simulink model "wheeled_balancer_model_simscape"  (R2024b)
settings: Solver=VariableStepAuto  StartTime=0.0  StopTime=3  FixedStep=0.001  MaxStep=0.0001  RelTol=1e-3  AbsTol=1e-3  EnableMultiTasking=on
StartFcn:
  | wheeled_balancer_model_simscape
values from neighbouring files (symbols this model uses):
  A = double(subs(Api,[g,M,m,b,l,I],[g_real,M_real,m_real,b_real,     l_real,I_real]))    [Scratchwork_cart.m]    (also in Scratchwork_pendulums.m = [0 1; a/l 0]; wheeled_balancer_model_simscape_script.m = double(subs(Asym,[g_sym,m_c_sym,m_sym,mu_c_sym,l_sym,J_sym,r)
  B = double(subs(Bpi,[g,M,m,b,l,I],[g_real,M_real,m_real,b_real,     l_real,I_real]))    [Scratchwork_cart.m]    (also in Scratchwork_pendulums.m = [0; 1/(m*l^2)]; wheeled_balancer_model_simscape_script.m = double(subs(Bsym,[g_sym,m_c_sym,m_sym,mu_c_sym,l_sym,J_sym,r)
  C = [1 0 0 0; 0 0 1 0]    [Scratchwork_cart.m]    (also in Scratchwork_pendulums.m = [1 0]; wheeled_balancer_model_simscape_script.m = [1 0 0 0; 0 0 0 1])
  C2 = [1 0]    [wheeled_balancer_model_simscape_script.m]
  g = 9.81    [wheeled_balancer_model_simscape_script.m]
  J = (I_motor + I_bump + I_batt + I_cb)    (= 0.000441007536814)    [wheeled_balancer_model_simscape_script.m]
  K = acker(A,B,p)    [Scratchwork_cart.m]    (also in Scratchwork_pendulums.m = acker(A,B,poles); wheeled_balancer_model_simscape_script.m = acker(Abar, Bbar, pc_control), Ks = K(1:end-1))
  Ki = K(end)    [wheeled_balancer_model_simscape_script.m]
  Ks = K(1:end-1), Ki = K(end),    [wheeled_balancer_model_simscape_script.m]
  L = place(A',C',pc_observer)'    [wheeled_balancer_model_simscape_script.m]
  l = .1    (= 0.1)    [Scratchwork_pendulums.m]    (also in wheeled_balancer_model_simscape_script.m = CM_rot)
  m = 1    [Scratchwork_pendulums.m]    (also in wheeled_balancer_model_simscape_script.m = 0.2983)
  m_c = (m_wheels)    (= 0.0397)    [wheeled_balancer_model_simscape_script.m]
  mu_c = 0.02    [wheeled_balancer_model_simscape_script.m]
  r = 0.01    [Scratchwork_pendulums.m]    (also in wheeled_balancer_model_simscape_script.m = 0.04)
  T = 1/100    (= 0.01)    [wheeled_balancer_model_simscape_script.m]
  theta_init = 0    [wheeled_balancer_model_simscape_script.m]
undefined symbols (not defined in the file or in its folder): Cd, G, H, X, Y, Z
libraries: sm_lib x8, nesl_utility x6
settings Model: Creator=teowi  LastModifiedBy=teowi
settings SolverCC: AutoScaleAbsTol=off  AlgebraicLoopSolver=TrustRegion  MaxZcPerStep=1
settings DataIOCC: LimitDataPoints=on  MaxDataPoints=10000
settings OptimizationCC: ReuseModelBlockBuffer=off  LifeSpan=inf
settings DebuggingCC: UnconnectedInputMsg=warning  UnconnectedOutputMsg=warning  UnconnectedLineMsg=warning  AllowSymbolicDim=off  SubsystemReferenceDiagnosticForUnitTest=warning  SFUnexpectedBacktrackingDiag=warning  SFNoUnconditionalDefaultTransitionDiag=warning  SFExecutionAtInitializationDiag=none  ArithmeticOperatorsInVariantConditions=warning
settings ModelReferenceCC: EnableRefExpFcnMdlSchedulingChecks=on
settings SFSimCC: SimUseLocalCustomCode=off  CustomCodeUndefinedFunction=UseInterfaceOnly
settings RTWCC: RTWUseLocalCustomCode=off  GPUComputeCapability=3.5  DLArmComputeVersion=19.05
settings CodeAppCC: StateflowObjectComments=on
settings GRTTargetCC: TargetLangStandard=C89/C90 (ANSI)
settings ConfigComp: CovMetricSettings=dw  CovSaveCumulativeToWorkspaceVar=on  CovSaveSingleToWorkspaceVar=on  CovExternalEMLEnable=off  CovSFcnEnable=off
settings SimscapeCC: SimscapeLogType=all  SimscapeLogSimulationStatistics=on  SimscapeLogDataHistory=10000

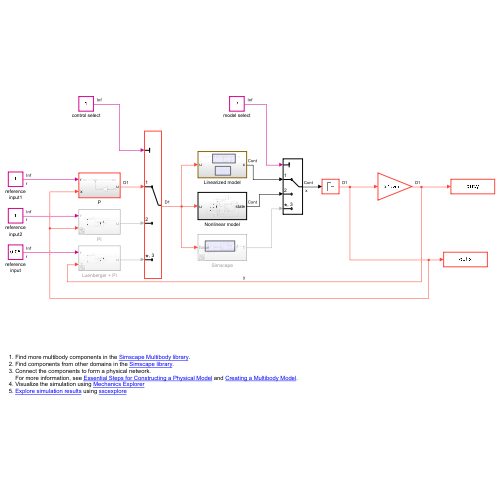
[thumbnail: Simulink's stored preview of the top-level diagram]
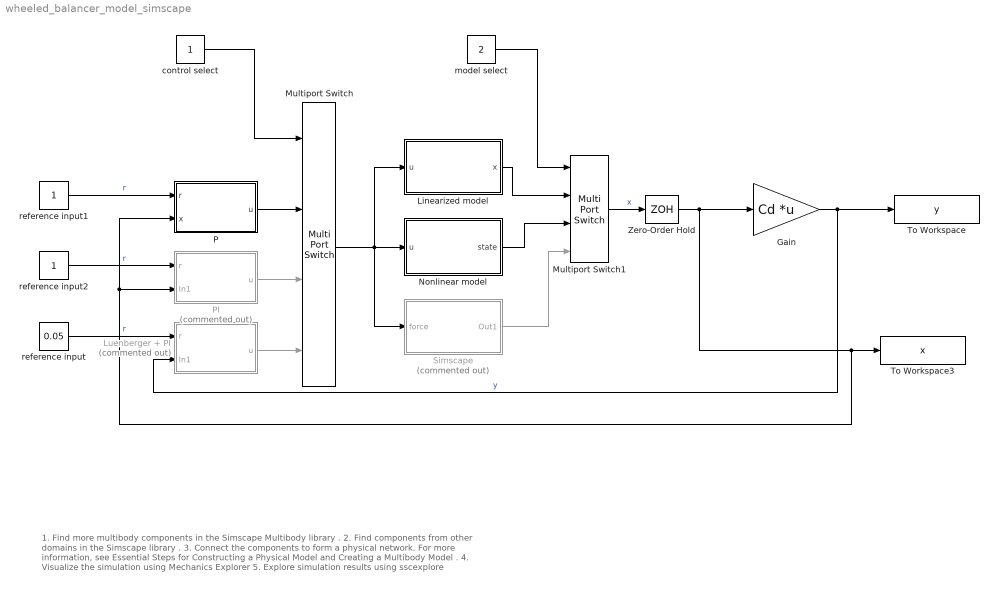
== system wheeled_balancer_model_simscape ==
  note: 1. Find more multibody components in the Simscape Multibody library .
      | 2. Find components from other domains in the Simscape library .
      | 3. Connect the components to form a physical network.
      | For more information, see Essential Steps for Constructing a Physical Model and Creating a Multibody Model .
      | 4. Visualize the simulation using Mechanics Explorer
      | 5. Explore simulation results using sscexplore
  Gain : Gain  Gain=Cd  Multiplication=Matrix(K*u) (u vector)
  Linearized model : Subsystem
  Luenberger + PI : Subsystem  Commented=on
  Multiport Switch : MultiPortSwitch  SaturateOnIntegerOverflow=off  InputSameDT=off
  Multiport Switch1 : MultiPortSwitch  SaturateOnIntegerOverflow=off  InputSameDT=off
  Nonlinear model : Subsystem
  P : Subsystem
  PI : Subsystem  Commented=on
  Simscape : Subsystem  Commented=on
  To Workspace : ToWorkspace  VariableName=y  SaveFormat=Timeseries  SampleTime=-1
  To Workspace3 : ToWorkspace  VariableName=x  SaveFormat=Timeseries  SampleTime=-1
  Zero-Order Hold : ZeroOrderHold  SampleTime=T
  control select : Constant
  model select : Constant  Value=2
  reference input : Constant  Value=0.05
  reference input1 : Constant
  reference input2 : Constant
  wires:
  Gain/1 -> To Workspace/1, Luenberger + PI/2(In1)  "y"
  Multiport Switch1/1 -> Zero-Order Hold/1  "x"
  control select/1 -> Multiport Switch/1
  Luenberger + PI/1(u) -> Multiport Switch/4
  reference input/1 -> Luenberger + PI/1(r)  "r"
  PI/1(u) -> Multiport Switch/3
  P/1(u) -> Multiport Switch/2
  reference input1/1 -> P/1(r)  "r"
  reference input2/1 -> PI/1(r)  "r"
  Multiport Switch/1 -> Simscape/1(force), Nonlinear model/1(u), Linearized model/1(u)
  Simscape/1(Out1) -> Multiport Switch1/4
  Linearized model/1(x) -> Multiport Switch1/2
  model select/1 -> Multiport Switch1/1
  Nonlinear model/1(state) -> Multiport Switch1/3
  Zero-Order Hold/1 -> To Workspace3/1, PI/2(In1), P/2(x), Gain/1

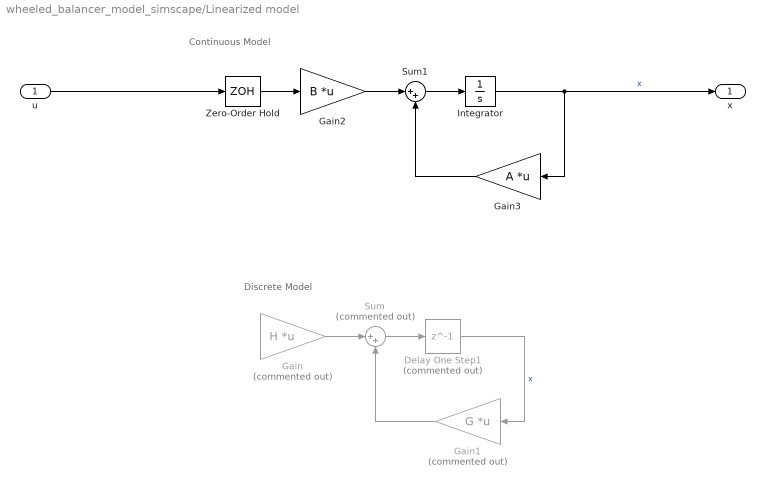
== system wheeled_balancer_model_simscape/Linearized model ==
  note: Discrete Model
  note: Continuous Model
  u : Inport
  Delay One Step1 : Delay  Commented=on  DelayLength=1  SampleTime=T
  Gain : Gain  Commented=on  Gain=H  Multiplication=Matrix(K*u) (u vector)
  Gain1 : Gain  Commented=on  Gain=G  Multiplication=Matrix(K*u) (u vector)
  Gain2 : Gain  Gain=B  Multiplication=Matrix(K*u) (u vector)
  Gain3 : Gain  Gain=A  Multiplication=Matrix(K*u) (u vector)
  Integrator : Integrator
  Sum : Sum  Commented=on  Inputs=|++
  Sum1 : Sum  Inputs=|++
  Zero-Order Hold : ZeroOrderHold  SampleTime=-1
  x : Outport
  wires:
  Sum/1 -> Delay One Step1/1
  Delay One Step1/1 -> Gain1/1  "x"
  Gain/1 -> Sum/1
  Gain1/1 -> Sum/2
  Integrator/1 -> Gain3/1, x/1  "x"
  Gain2/1 -> Sum1/1
  Sum1/1 -> Integrator/1
  Gain3/1 -> Sum1/2
  Zero-Order Hold/1 -> Gain2/1
  u/1 -> Zero-Order Hold/1

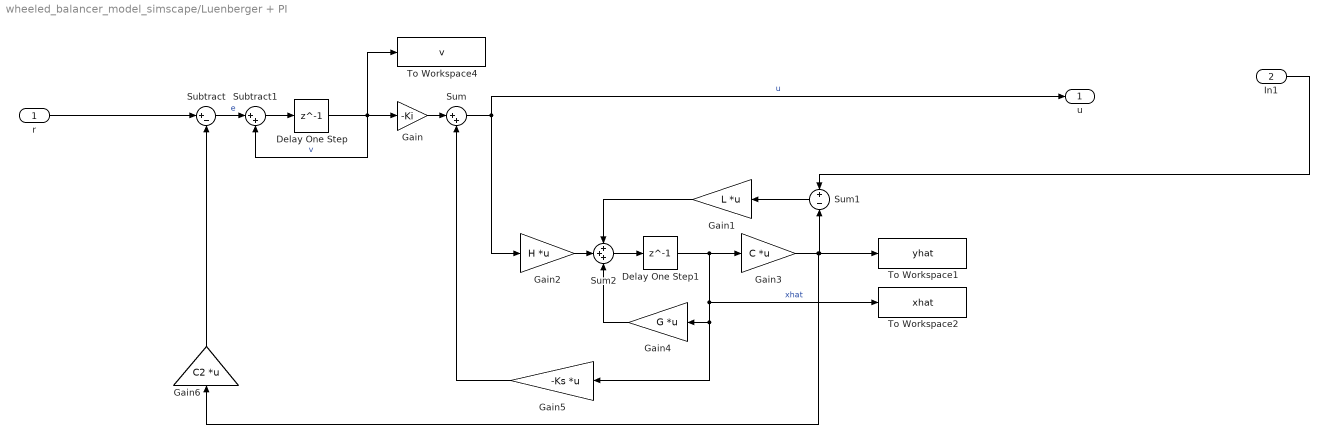
== system wheeled_balancer_model_simscape/Luenberger + PI ==
  r : Inport
  In1 : Inport  Port=2
  Delay One Step : Delay  DelayLength=1  SampleTime=T
  Delay One Step1 : Delay  DelayLength=1  SampleTime=T
  Gain : Gain  Gain=-Ki
  Gain1 : Gain  Gain=L  Multiplication=Matrix(K*u) (u vector)
  Gain2 : Gain  Gain=H  Multiplication=Matrix(K*u) (u vector)
  Gain3 : Gain  Gain=C  Multiplication=Matrix(K*u) (u vector)
  Gain4 : Gain  Gain=G  Multiplication=Matrix(K*u) (u vector)
  Gain5 : Gain  Gain=-Ks  Multiplication=Matrix(K*u) (u vector)
  Gain6 : Gain  Gain=C2  Multiplication=Matrix(K*u) (u vector)
  Subtract : Sum  Inputs=|+-
  Subtract1 : Sum  Inputs=|++
  Sum : Sum  Inputs=|++
  Sum1 : Sum  Inputs=+|-
  Sum2 : Sum  Inputs=+++
  To Workspace1 : ToWorkspace  VariableName=yhat  SaveFormat=Timeseries  SampleTime=-1
  To Workspace2 : ToWorkspace  VariableName=xhat  SaveFormat=Timeseries  SampleTime=-1
  To Workspace4 : ToWorkspace  VariableName=v  SaveFormat=Timeseries  SampleTime=-1
  u : Outport
  wires:
  Delay One Step1/1 -> Gain4/1, Gain5/1, To Workspace2/1, Gain3/1  "xhat"
  Sum/1 -> u/1, Gain2/1  "u"
  r/1 -> Subtract/1
  Delay One Step/1 -> To Workspace4/1, Gain/1, Subtract1/2  "v"
  Gain5/1 -> Sum/2
  Subtract/1 -> Subtract1/1  "e"
  Gain/1 -> Sum/1
  Gain1/1 -> Sum2/1
  Gain3/1 -> To Workspace1/1, Sum1/2, Gain6/1
  Gain2/1 -> Sum2/2
  Sum1/1 -> Gain1/1
  Gain6/1 -> Subtract/2
  Subtract1/1 -> Delay One Step/1
  Gain4/1 -> Sum2/3
  Sum2/1 -> Delay One Step1/1
  In1/1 -> Sum1/1

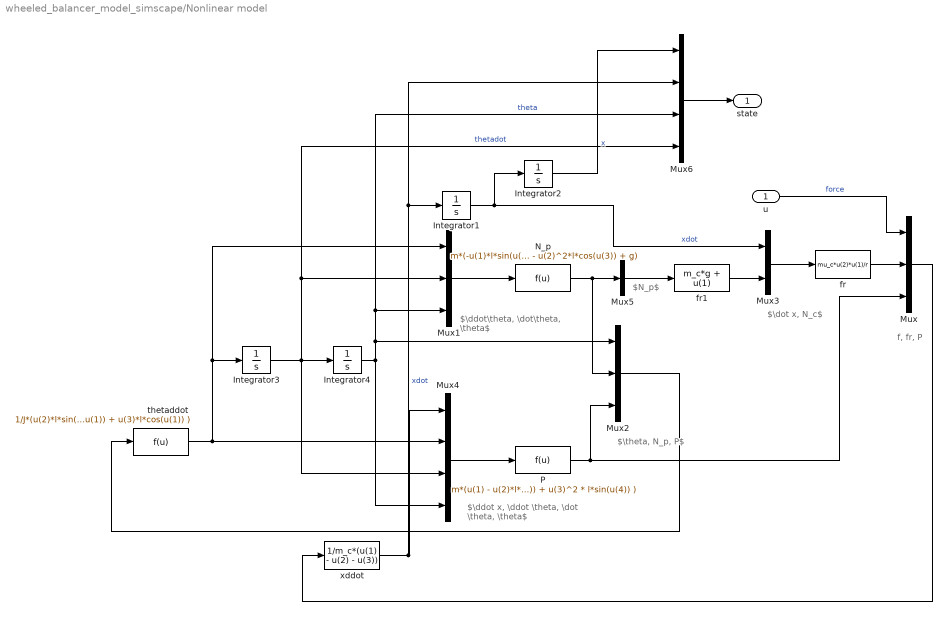
== system wheeled_balancer_model_simscape/Nonlinear model ==
  note: f, fr, P
  note: $\theta, N_p, P$
  note: $\dot x, N_c$
  note: $N_p$
  note: $\ddot\theta, \dot\theta, \theta$
  note: $\ddot x, \ddot \theta, \dot \theta, \theta$
  u : Inport
  Integrator1 : Integrator
  Integrator2 : Integrator
  Integrator3 : Integrator
  Integrator4 : Integrator  InitialCondition=theta_init
  Mux : Mux  Inputs=3
  Mux1 : Mux  Inputs=3
  Mux2 : Mux  Inputs=3
  Mux3 : Mux  Inputs=2
  Mux4 : Mux
  Mux5 : Mux  Inputs=1
  Mux6 : Mux
  N_p : Fcn  Expr=m*(-u(1)*l*sin(u(3)) - u(2)^2*l*cos(u(3)) + g)
  P : Fcn  Expr=m*(u(1) - u(2)*l*cos(u(4)) + u(3)^2 * l*sin(u(4)) )
  fr : Fcn  Expr=mu_c*u(2)*u(1)/r
  fr1 : Fcn  Expr=m_c*g + u(1)
  thetaddot : Fcn  Expr=1/J*(u(2)*l*sin(u(1)) + u(3)*l*cos(u(1)) )
  xddot : Fcn  Expr=1/m_c*(u(1) - u(2) - u(3))
  state : Outport
  wires:
  Mux2/1 -> thetaddot/1
  Integrator1/1 -> Integrator2/1, Mux3/1  "xdot"
  xddot/1 -> Mux6/2, Integrator1/1, Mux4/1  "xdot"
  thetaddot/1 -> Mux1/1, Integrator3/1, Mux4/2
  Integrator4/1 -> Mux2/1, Mux6/3, Mux1/3, Mux4/4  "theta"
  Integrator3/1 -> Mux4/3, Integrator4/1, Mux6/4, Mux1/2  "thetadot"
  Mux4/1 -> P/1
  Mux1/1 -> N_p/1
  N_p/1 -> Mux5/1, Mux2/2
  fr1/1 -> Mux3/2
  P/1 -> Mux/3, Mux2/3
  Mux5/1 -> fr1/1
  Mux/1 -> xddot/1
  Mux3/1 -> fr/1
  u/1 -> Mux/1  "force"
  fr/1 -> Mux/2
  Integrator2/1 -> Mux6/1  "x"
  Mux6/1 -> state/1

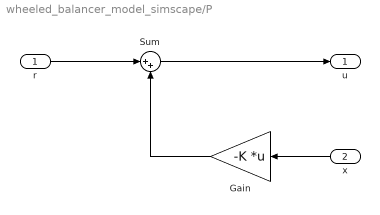
== system wheeled_balancer_model_simscape/P ==
  r : Inport
  x : Inport  Port=2
  Gain : Gain  Gain=-K  Multiplication=Matrix(K*u) (u vector)
  Sum : Sum  Inputs=|++
  u : Outport
  wires:
  r/1 -> Sum/1
  x/1 -> Gain/1
  Gain/1 -> Sum/2
  Sum/1 -> u/1

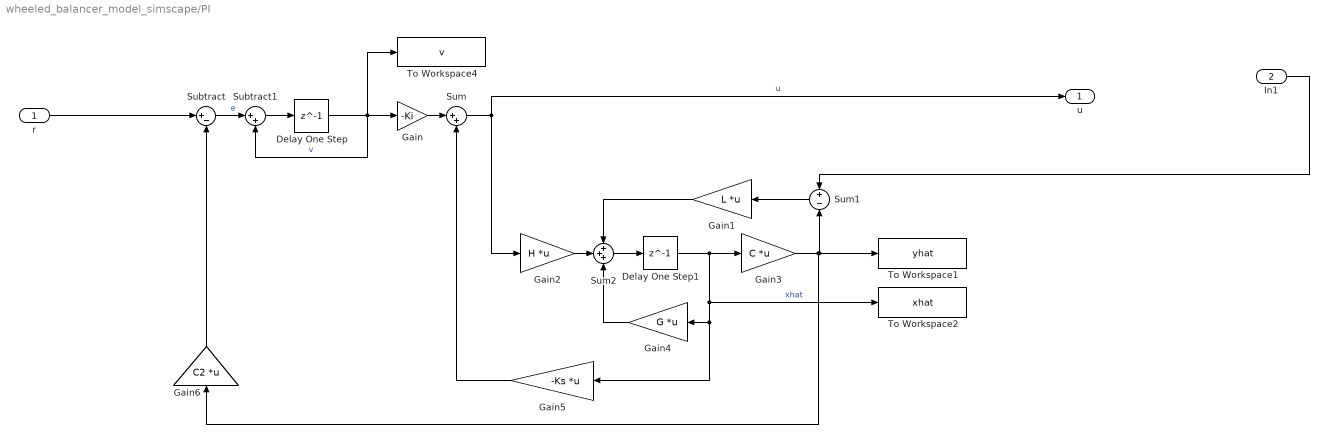
== system wheeled_balancer_model_simscape/PI ==
  r : Inport
  In1 : Inport  Port=2
  Delay One Step : Delay  DelayLength=1  SampleTime=T
  Delay One Step1 : Delay  DelayLength=1  SampleTime=T
  Gain : Gain  Gain=-Ki
  Gain1 : Gain  Gain=L  Multiplication=Matrix(K*u) (u vector)
  Gain2 : Gain  Gain=H  Multiplication=Matrix(K*u) (u vector)
  Gain3 : Gain  Gain=C  Multiplication=Matrix(K*u) (u vector)
  Gain4 : Gain  Gain=G  Multiplication=Matrix(K*u) (u vector)
  Gain5 : Gain  Gain=-Ks  Multiplication=Matrix(K*u) (u vector)
  Gain6 : Gain  Gain=C2  Multiplication=Matrix(K*u) (u vector)
  Subtract : Sum  Inputs=|+-
  Subtract1 : Sum  Inputs=|++
  Sum : Sum  Inputs=|++
  Sum1 : Sum  Inputs=+|-
  Sum2 : Sum  Inputs=+++
  To Workspace1 : ToWorkspace  VariableName=yhat  SaveFormat=Timeseries  SampleTime=-1
  To Workspace2 : ToWorkspace  VariableName=xhat  SaveFormat=Timeseries  SampleTime=-1
  To Workspace4 : ToWorkspace  VariableName=v  SaveFormat=Timeseries  SampleTime=-1
  u : Outport
  wires:
  Delay One Step1/1 -> Gain4/1, Gain5/1, To Workspace2/1, Gain3/1  "xhat"
  Sum/1 -> u/1, Gain2/1  "u"
  r/1 -> Subtract/1
  Delay One Step/1 -> To Workspace4/1, Gain/1, Subtract1/2  "v"
  Gain5/1 -> Sum/2
  Subtract/1 -> Subtract1/1  "e"
  Gain/1 -> Sum/1
  Gain1/1 -> Sum2/1
  Gain3/1 -> To Workspace1/1, Sum1/2, Gain6/1
  Gain2/1 -> Sum2/2
  Sum1/1 -> Gain1/1
  Gain6/1 -> Subtract/2
  Subtract1/1 -> Delay One Step/1
  Gain4/1 -> Sum2/3
  Sum2/1 -> Delay One Step1/1
  In1/1 -> Sum1/1

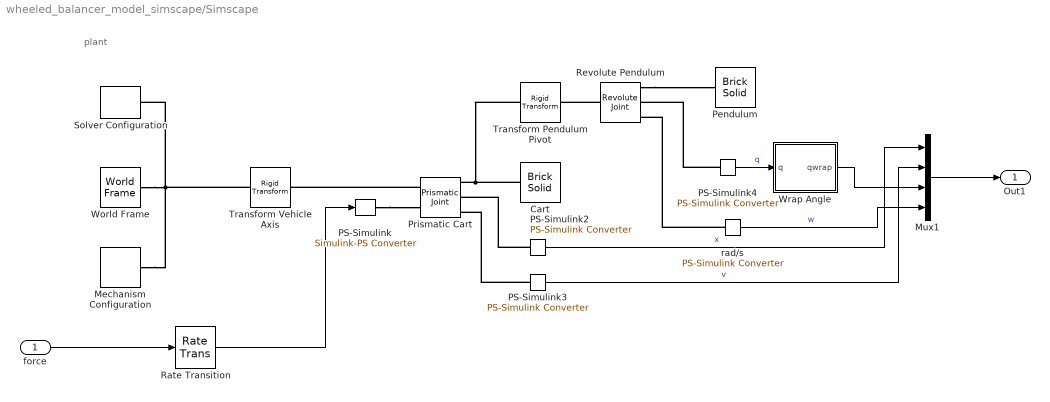
== system wheeled_balancer_model_simscape/Simscape ==
  note: plant
  force : Inport
  Cart : sm_lib/Body Elements/Brick Solid  BrickDimensions=[0.02 0.04 0.06]  BrickDimensionsUnits=m  ExportEntireGeometry=off  InertiaType=PointMass  BasedOnType=Density  Density=1000  DensityUnits=kg/m^3  Mass=m_c  MassUnits=kg  CenterOfMass=[0 0 0]  CenterOfMassUnits=m  MomentsOfInertia=[1 1 1]  MomentsOfInertiaUnits=kg*m^2  ProductsOfInertia=[0 0 0]  ProductsOfInertiaUnits=kg*m^2  GraphicType=FromGeometry  MarkerShape=Sphere  MarkerSize=10  GraphicVisPropType=SimpleVisualProperties  GraphicDiffuseColor=[0.8 0.45 0]  GraphicOpacity=1.0  GraphicSpecularColor=[0.5 0.5 0.5 1.0]  GraphicAmbientColor=[0.15 0.15 0.15 1.0]  GraphicEmissiveColor=[0.0 0.0 0.0 1.0]  GraphicShininess=75  DoExposeReferenceFrame=on  SerializedFrames=<Frames/>
  Mechanism Configuration : sm_lib/Utilities/Mechanism Configuration  UniformGravity=Constant  GravityVector=[0 0 -g]  GravityVectorUnits=m/s^2  LinearizationDelta=0.001  JointModeTransitionNonlinearIterations=2
  Mux1 : Mux
  PS-Simulink : nesl_utility/Simulink-PS Converter  PhysicalDomain=network_engine_domain  SubClassName=ps_input  LeftPortType=input  RightPortType=output  PseudoPeriodic=off  Frequencies=[]  NoiseDistribution=none  NoiseParameters=[]  Unit=N  AffineConversion=off  FilteringAndDerivatives=provide  SimscapeFilterOrder=1  InputFilterTimeConstant=0.001  UdotUserProvided=0
  PS-Simulink2 : nesl_utility/PS-Simulink Converter  PhysicalDomain=network_engine_domain  SubClassName=ps_output  LeftPortType=input  RightPortType=output  PseudoPeriodic=off  Frequencies=[]  VectorFormat=inherit  Unit=m  AffineConversion=off
  PS-Simulink3 : nesl_utility/PS-Simulink Converter  PhysicalDomain=network_engine_domain  SubClassName=ps_output  LeftPortType=input  RightPortType=output  PseudoPeriodic=off  Frequencies=[]  VectorFormat=inherit  Unit=m/s  AffineConversion=off
  PS-Simulink4 : nesl_utility/PS-Simulink Converter  PhysicalDomain=network_engine_domain  SubClassName=ps_output  LeftPortType=input  RightPortType=output  PseudoPeriodic=off  Frequencies=[]  VectorFormat=inherit  Unit=rad  AffineConversion=off
  Pendulum : sm_lib/Body Elements/Brick Solid  BrickDimensions=[l*2 0.04 0.02]  BrickDimensionsUnits=m  ExportEntireGeometry=off  InertiaType=PointMass  BasedOnType=Density  Density=1000  DensityUnits=kg/m^3  Mass=m  MassUnits=kg  CenterOfMass=[0 0 0]  CenterOfMassUnits=m  MomentsOfInertia=[1 1 1]  MomentsOfInertiaUnits=kg*m^2  ProductsOfInertia=[0 0 0]  ProductsOfInertiaUnits=kg*m^2  GraphicType=FromGeometry  MarkerShape=Sphere  MarkerSize=10  GraphicVisPropType=SimpleVisualProperties  GraphicDiffuseColor=[0.25 0.4 0.7]  GraphicOpacity=1  GraphicSpecularColor=[0.5 0.5 0.5 1.0]  GraphicAmbientColor=[0.15 0.15 0.15 1.0]  GraphicEmissiveColor=[0.0 0.0 0.0 1.0]  GraphicShininess=75  DoExposeReferenceFrame=off  SerializedFrames=<Frames><Frame><Id>Frame1</Id><Value><Name>B</Name><Origin><Source>GeometricFeature</Source><FeatureName>+x surface</FeatureName></Origin><PrimaryAxis><DefinedDirection>+Z</DefinedDirection><Source>ReferenceFrame</Source><SourceDirection>+Z</SourceDirection><FeatureName></FeatureName></PrimaryAxis><SecondaryAxis><DefinedDirection>+X</DefinedDirection><Source>ReferenceFrame</Source><SourceDirection>+X</SourceDirection><FeatureName></FeatureName></SecondaryAxis></Value></Frame></Frames>
  Prismatic Cart : sm_lib/Joints/Prismatic Joint  JointMode=Normal  CompositeWrenchDir=FollowerOnBase  CompositeWrenchFrame=BaseFrame  SenseConstraintForce=off  SenseConstraintTorque=off  SenseTotalForce=off  SenseTotalTorque=off  PositionTargetSpecify=off  PositionTargetPriority=High  PositionTargetValue=0  PositionTargetValueUnits=m  VelocityTargetSpecify=off  VelocityTargetPriority=High  VelocityTargetValue=0  VelocityTargetValueUnits=m/s  EquilibriumPosition=0  EquilibriumPositionUnits=m  SpringStiffness=0  SpringStiffnessUnits=N/m  DampingCoefficient=mu_c*(m+m_c)*g/r  DampingCoefficientUnits=N/(m/s)  LowerLimitSpecify=off  LowerLimitBound=-1  LowerLimitBoundUnits=m  LowerLimitStiffness=1e6  LowerLimitStiffnessUnits=N/m  LowerLimitDamping=1e3  LowerLimitDampingUnits=N/(m/s)  LowerLimitTransitionRegionWidth=1e-4  LowerLimitTransitionRegionWidthUnits=m  UpperLimitSpecify=off  UpperLimitBound=1  UpperLimitBoundUnits=m  UpperLimitStiffness=1e6  UpperLimitStiffnessUnits=N/m  UpperLimitDamping=1e3  UpperLimitDampingUnits=N/(m/s)  UpperLimitTransitionRegionWidth=1e-4  UpperLimitTransitionRegionWidthUnits=m  TorqueActuationMode=InputTorque  MotionActuationMode=ComputedMotion  SensePosition=on  SenseVelocity=on  SenseAcceleration=off  SenseTorqueForce=off  SenseLowerLimitTorqueForce=off  SenseUpperLimitTorqueForce=off
  Rate Transition : RateTransition
  Revolute Pendulum : sm_lib/Joints/Revolute Joint  JointMode=Normal  CompositeWrenchDir=FollowerOnBase  CompositeWrenchFrame=BaseFrame  SenseConstraintForce=off  SenseConstraintTorque=off  SenseTotalForce=off  SenseTotalTorque=off  PositionTargetSpecify=off  PositionTargetPriority=High  PositionTargetValue=0  PositionTargetValueUnits=deg  VelocityTargetSpecify=off  VelocityTargetPriority=High  VelocityTargetValue=0  VelocityTargetValueUnits=deg/s  EquilibriumPosition=0  EquilibriumPositionUnits=deg  SpringStiffness=0  SpringStiffnessUnits=N*m/deg  DampingCoefficient=0  DampingCoefficientUnits=N*m/(deg/s)  LowerLimitSpecify=off  LowerLimitBound=-90  LowerLimitBoundUnits=deg  LowerLimitStiffness=1e4  LowerLimitStiffnessUnits=N*m/deg  LowerLimitDamping=10  LowerLimitDampingUnits=N*m/(deg/s)  LowerLimitTransitionRegionWidth=0.1  LowerLimitTransitionRegionWidthUnits=deg  UpperLimitSpecify=off  UpperLimitBound=90  UpperLimitBoundUnits=deg  UpperLimitStiffness=1e4  UpperLimitStiffnessUnits=N*m/deg  UpperLimitDamping=10  UpperLimitDampingUnits=N*m/(deg/s)  UpperLimitTransitionRegionWidth=0.1  UpperLimitTransitionRegionWidthUnits=deg  TorqueActuationMode=NoTorque  MotionActuationMode=ComputedMotion  SensePosition=on  SenseVelocity=on  SenseAcceleration=off  SenseTorqueForce=off  SenseLowerLimitTorqueForce=off  SenseUpperLimitTorqueForce=off
  Solver Configuration : nesl_utility/Solver Configuration  PhysicalDomain=network_engine_domain  SubClassName=solver  LeftPortType=input  RightPortType=generic  Tones=[]  Harmonics=[]  SimulateNoise=off  Profile=off  UseLocalSampling=off  EnableSwitchedLinearOptims=on  FrequencyDomain=off  UseCCode=off  RelTol=0.001  AbsTol=1e-06  MinStep=1e-09  ToWorkspace=off  RevertToSquareIcSolve=off  NumHomotopyIterations=100  PhasorMode=off  PhasorModeNumHarmonics=1  ConsistencySolver=NEWTON_XTOL_AFTER_FTOL  IndexReductionMethod=DerivativeReplacement  DoDC=off  ResidualTolerance=1e-09  ConsistencyTolSource=GLOBAL  ConsistencyAbsTol=0.001  ConsistencyRelTol=0.001  ConsistencyTolFactor=0.001  UseLocalSolver=off  LocalSolverChoice=NE_BACKWARD_EULER_ADVANCER  ResolveIndetEquations=on  FunctionEvalNumThread=1  LocalSolverSampleTime=0.0001  DoFixedCost=off  MaxNonlinIter=3  MaxModeIter=2  ComputeImpulses=off  ImpulseIterations=2  LinearAlgebra=Sparse  LinearAlgebraNumThread=0  EquationFormulation=NE_TIME_EF  DelaysMemoryBudget=1024  AutomaticFiltering=on  FilteringTimeConstant=0.001  PartitionStorageMethod=AS_NEEDED  PartitionMemoryBudget=1024  PartitionMethod=FAST  MultibodyUseLocalSolver=off  MultibodyLocalSolverChoice=ODE1  MultibodyLocalSolverSampleTime=0.001
  Transform Pendulum Pivot : sm_lib/Frames and Transforms/Rigid Transform  RotationMethod=StandardAxis  FollAlignAxisA=+X  BaseAlignAxisA=+Y  FollAlignAxisB=+Y  BaseAlignAxisB=+Z  RotationStandardAxis=+X  RotationAngle=-90  RotationAngleUnits=deg  RotationArbitraryAxis=[0 0 1]  RotationSequenceAxes=FollowerAxes  RotationSequence=XYX  RotationSequenceAngles=[0 0 0]  RotationSequenceAnglesUnits=deg  RotationMatrix=[1 0 0; 0 1 0; 0 0 1]  Quaternion=[1 0 0 0]  TranslationMethod=None  TranslationCartesianOffset=[0 0 0]  TranslationCartesianOffsetUnits=m  TranslationStandardAxis=+Z  TranslationStandardOffset=0  TranslationStandardOffsetUnits=m  TranslationROffset=0  TranslationROffsetUnits=m  TranslationThetaOffset=0  TranslationThetaOffsetUnits=deg  TranslationZOffset=0  TranslationZOffsetUnits=m
  Transform Vehicle Axis : sm_lib/Frames and Transforms/Rigid Transform  RotationMethod=StandardAxis  FollAlignAxisA=+X  BaseAlignAxisA=+Y  FollAlignAxisB=+Y  BaseAlignAxisB=+Z  RotationStandardAxis=+Y  RotationAngle=90  RotationAngleUnits=deg  RotationArbitraryAxis=[0 0 1]  RotationSequenceAxes=FollowerAxes  RotationSequence=XYX  RotationSequenceAngles=[0 0 0]  RotationSequenceAnglesUnits=deg  RotationMatrix=[1 0 0; 0 1 0; 0 0 1]  Quaternion=[1 0 0 0]  TranslationMethod=None  TranslationCartesianOffset=[0 0 0]  TranslationCartesianOffsetUnits=m  TranslationStandardAxis=+Z  TranslationStandardOffset=0  TranslationStandardOffsetUnits=m  TranslationROffset=0  TranslationROffsetUnits=m  TranslationThetaOffset=0  TranslationThetaOffsetUnits=deg  TranslationZOffset=0  TranslationZOffsetUnits=m
  World Frame : sm_lib/Frames and Transforms/World Frame
  Wrap Angle : Subsystem
  rad/s : nesl_utility/PS-Simulink Converter  PhysicalDomain=network_engine_domain  SubClassName=ps_output  LeftPortType=input  RightPortType=output  PseudoPeriodic=off  Frequencies=[]  VectorFormat=inherit  Unit=rad/s  AffineConversion=off
  Out1 : Outport
  wires:
  Mux1/1 -> Out1/1
  force/1 -> Rate Transition/1
  Wrap Angle/1(qwrap) -> Mux1/3
  PS-Simulink2/1 -> Mux1/1  "x"
  PS-Simulink3/1 -> Mux1/2  "v"
  PS-Simulink4/1 -> Wrap Angle/1(q)  "q"
  rad/s/1 -> Mux1/4  "w"
  Rate Transition/1 -> PS-Simulink/1
  connections:
  PS-Simulink4/LConn1 -- Revolute Pendulum/RConn2
  rad/s/LConn1 -- Revolute Pendulum/RConn3
  Revolute Pendulum/RConn1 -- Pendulum/LConn1
  PS-Simulink/RConn1 -- Prismatic Cart/LConn2
  Prismatic Cart/LConn1 -- Transform Vehicle Axis/RConn1
  Cart/RConn1 -- Transform Pendulum Pivot/LConn1 -- Prismatic Cart/RConn1
  PS-Simulink2/LConn1 -- Prismatic Cart/RConn2
  PS-Simulink3/LConn1 -- Prismatic Cart/RConn3
  Revolute Pendulum/LConn1 -- Transform Pendulum Pivot/RConn1
  World Frame/RConn1 -- Transform Vehicle Axis/LConn1 -- Mechanism Configuration/RConn1 -- Solver Configuration/RConn1

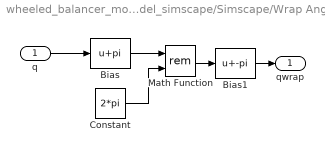
== system wheeled_balancer_model_simscape/Simscape/Wrap Angle ==
  q : Inport
  Bias : Bias  Bias=pi  SaturateOnIntegerOverflow=off
  Bias1 : Bias  Bias=-pi  SaturateOnIntegerOverflow=off
  Constant : Constant  Value=2*pi
  Math Function : Math  Operator=rem
  qwrap : Outport
  wires:
  q/1 -> Bias/1
  Bias/1 -> Math Function/1
  Constant/1 -> Math Function/2
  Math Function/1 -> Bias1/1
  Bias1/1 -> qwrap/1
